simulink model "Example_AswarmTriangleCallibration"  (R2023b)
settings: Solver=FixedStepAuto  StartTime=0.0  StopTime=1  FixedStep=0.1  RelTol=1e-3  EnableMultiTasking=on
undefined symbols (not defined in the file or in its folder): numtestpoint4, testpoint4
libraries: simulink x1
settings Model: Creator=damerius  LastModifiedBy=khalis
settings SolverCC: ConcurrentTasks=on  AlgebraicLoopSolver=TrustRegion  PositivePriorityOrder=on
settings DataIOCC: SaveOutput=off  SignalLogging=off  DSMLogging=off  SaveTime=off  ReturnWorkspaceOutputs=off
settings OptimizationCC: DefaultParameterBehavior=Inlined  ReuseModelBlockBuffer=off  ZeroExternalMemoryAtStartup=off  ZeroInternalMemoryAtStartup=off  SimCompilerOptimization=on
settings DebuggingCC: UnconnectedInputMsg=warning  UnconnectedOutputMsg=warning  UnconnectedLineMsg=warning
settings HardwareCC: ProdBitPerLong=64  ProdHWDeviceType=Intel->x86-64 (Linux 64)
settings ModelReferenceCC: EnableRefExpFcnMdlSchedulingChecks=on
settings SFSimCC: SimParseCustomCode=off  SimGenImportedTypeDefs=on  SimTargetLang=C++
settings RTWCC: GenCodeOnly=on  PackageGeneratedCodeAndArtifacts=on  PackageName=PackNGo  RTWVerbose=off  BuildConfiguration=Faster Runs  TargetLang=C++  DLArmComputeVersion=19.05
settings CodeAppCC: ForceParamTrailComments=on  MaxIdLength=95  MATLABSourceComments=on  UseSimReservedNames=on
settings GRTTargetCC: TargetLangStandard=C++11 (ISO)  GenerateFullHeader=off  MatFileLogging=off  CodeInterfacePackaging=C++ class

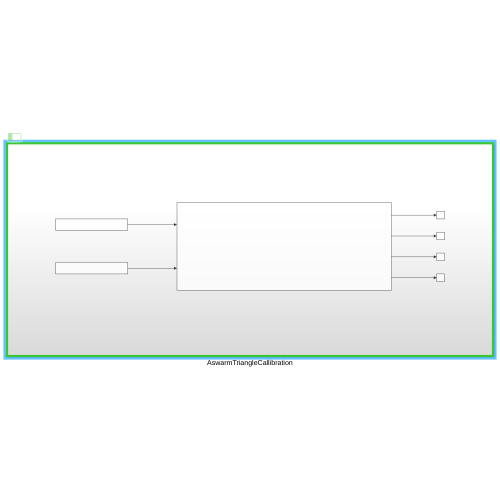
[thumbnail: Simulink's stored preview of the top-level diagram]
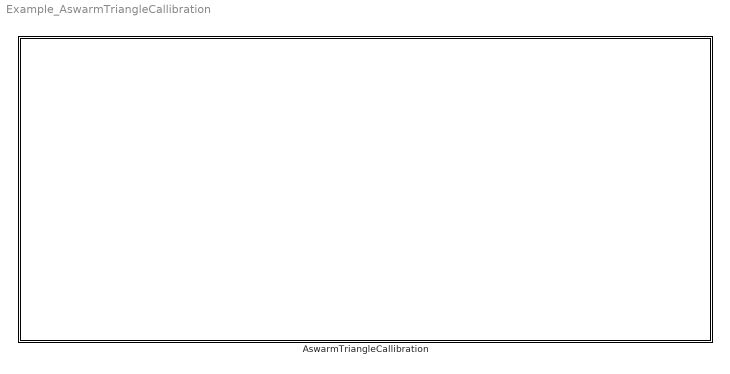
== system Example_AswarmTriangleCallibration ==
  AswarmTriangleCallibration : Subsystem  TreatAsAtomicUnit=on  ScheduleAs=Periodic partition  PartitionName=linedetector  SystemSampleTime=2

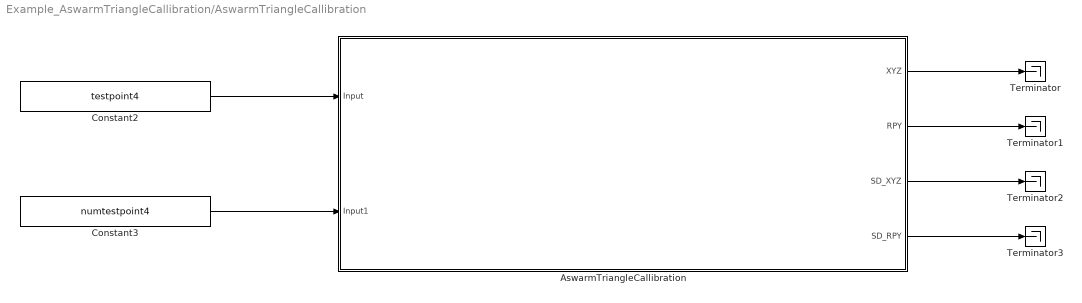
== system Example_AswarmTriangleCallibration/AswarmTriangleCallibration ==
  AswarmTriangleCallibration : Subsystem  ScheduleAs=Periodic partition  PartitionName=linedetector  SystemSampleTime=2  mask{Parameter1=0.1, Parameter2=1.0, Parameter3=500, Parameter4=256000, Parameter5=1.0, Parameter6=0.12, Parameter7=0.12, Parameter8=-2.0, Parameter9=-1.1, Parameter10=10.0, Parameter11=4.0, Parameter12=10.7703, Parameter13=90.0, Parameter14=21.80, Parameter15=68.20, Parameter16=0.001, Parameter17=0.001, Parameter18=2.0}
      mask prompts: Parameter1 "leafSize[m]:"; Parameter2 "clusterTolerance:"; Parameter3 "minClusterSize:"; Parameter4 "maxClusterSize:"; Parameter5 "radiusSearch[m]:"; Parameter6 "curvatureThresholdPlane:"; Parameter7 "curvatureThresholdCorner:"; Parameter8 "normalDistanceMin[m]:"; Parameter9 "normalDistanceMax[m]:"; Parameter10 "adjacentSide[m]:"; Parameter11 "oppositeSide[m]:"; Parameter12 "hypotenuse[m]:"; Parameter13 "adjacentAngle[°]:"; Parameter14 "oppositeAngle[°]:"; Parameter15 "vertexAngle[°]:"; Parameter16 "distanceTolerance[m]:"; Parameter17 "angleTolerance[°]:"; Parameter18 "searchRadius[m]:"
      mask DialogControl Container4 Prompt: Downsampling Parameter
      mask DialogControl Control2 Prompt: The size of the voxel grid for downsampling.
      mask DialogControl Container5 Prompt: Vehicle Clustering Parameter
      mask DialogControl Control3 Prompt: This algorithm will find nearest cluster as the vehicle cluster.
      mask DialogControl Container6 Prompt: Feature Extraction Parameter
      mask DialogControl Control4 Prompt: This algorithm will extract the plane and corner features.
      mask DialogControl Container9 Prompt: Plane Limit Parameter
      mask DialogControl Control5 Prompt: Sometime the vehicle surface plane is not visibile due to the object on the plane. Thus, to extract the surface plane only we need to apply passthrough filter in the plane normal.
      mask DialogControl Container10 Prompt: Ideal Triangle and Candidate Search Parameter:
      mask DialogControl Control7 Prompt: Ideal Right Triangle:
      mask DialogControl Control6 Prompt: This algorithm will find the best Right Triangle fit for the given input pointCloud.
      mask Display:
      | disp("Aswarm Triangle Callibration");
      | 
      | port_label('input',1,'inputCloud');
      | port_label('input',2,'numInputCloud');
  Constant2 : Constant  Value=testpoint4  OutDataTypeStr=single
  Constant3 : Constant  Value=numtestpoint4  OutDataTypeStr=uint32
  Terminator{,1..3} (4 alike) : Terminator
  wires:
  Constant2/1 -> AswarmTriangleCallibration/1(Input)
  Constant3/1 -> AswarmTriangleCallibration/2(Input1)
  AswarmTriangleCallibration/1(XYZ) -> Terminator/1
  AswarmTriangleCallibration/2(RPY) -> Terminator1/1
  AswarmTriangleCallibration/3(SD_XYZ) -> Terminator2/1
  AswarmTriangleCallibration/4(SD_RPY) -> Terminator3/1

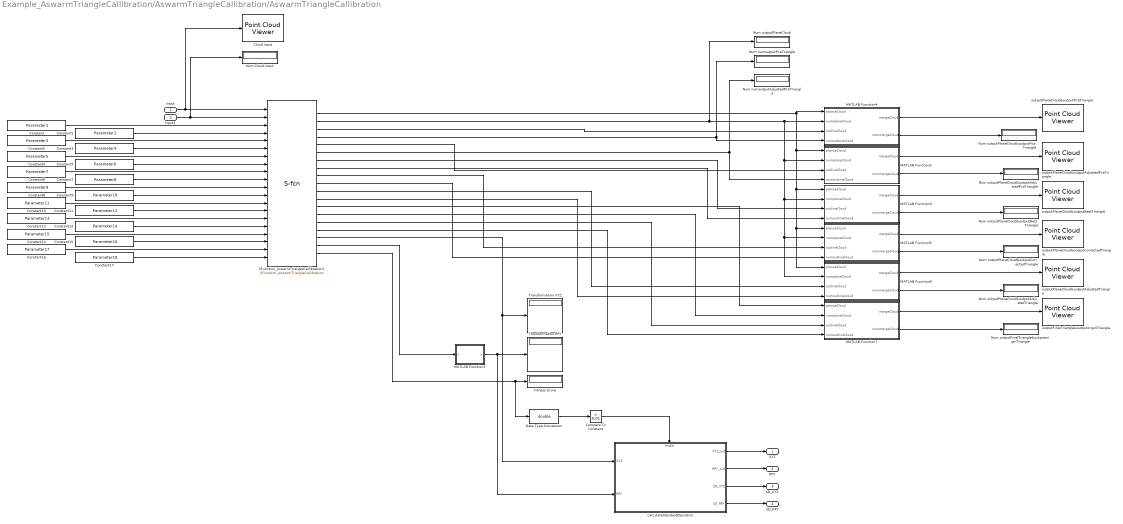
== system Example_AswarmTriangleCallibration/AswarmTriangleCallibration/AswarmTriangleCallibration ==
  Input : Inport
  Input1 : Inport  Port=2
  Cloud Input : PointCloudViewer  FigPos=[9 1380 570 1291]
  Compare To Constant : simulink/Logic and Bit Operations/Compare To Constant  relop=<  const=0.01  OutDataTypeStr=boolean
  Constant : Constant  Value=Parameter1  OutDataTypeStr=double
  Constant1 : Constant  Value=Parameter2  OutDataTypeStr=double
  Constant10 : Constant  Value=Parameter11  OutDataTypeStr=double
  Constant11 : Constant  Value=Parameter12  OutDataTypeStr=double
  Constant12 : Constant  Value=Parameter13  OutDataTypeStr=double
  Constant13 : Constant  Value=Parameter14  OutDataTypeStr=double
  Constant14 : Constant  Value=Parameter15  OutDataTypeStr=double
  Constant15 : Constant  Value=Parameter16  OutDataTypeStr=double
  Constant16 : Constant  Value=Parameter17  OutDataTypeStr=double
  Constant17 : Constant  Value=Parameter18  OutDataTypeStr=double
  Constant2 : Constant  Value=Parameter3  OutDataTypeStr=uint32
  Constant3 : Constant  Value=Parameter4  OutDataTypeStr=uint32
  Constant4 : Constant  Value=Parameter5  OutDataTypeStr=double
  Constant5 : Constant  Value=Parameter6  OutDataTypeStr=double
  Constant6 : Constant  Value=Parameter7  OutDataTypeStr=double
  Constant7 : Constant  Value=Parameter8  OutDataTypeStr=double
  Constant8 : Constant  Value=Parameter9  OutDataTypeStr=double
  Constant9 : Constant  Value=Parameter10  OutDataTypeStr=double
  Data Type Conversion : DataTypeConversion  OutDataTypeStr=double  SaturateOnIntegerOverflow=off  RndMeth=Floor
  Fitness Score : Display
  MATLAB Function1 : MATLAB Function  TreatAsAtomicUnit=on
  MATLAB Function2 : MATLAB Function  TreatAsAtomicUnit=on
  MATLAB Function3 : MATLAB Function  TreatAsAtomicUnit=on
  MATLAB Function4 : MATLAB Function  TreatAsAtomicUnit=on
  MATLAB Function5 : MATLAB Function  TreatAsAtomicUnit=on
  MATLAB Function6 : MATLAB Function  TreatAsAtomicUnit=on
  MATLAB Function7 : MATLAB Function  TreatAsAtomicUnit=on
  Num Cloud Input : Display
  Num numoutputAdjustedPcaTriangle : Display
  Num numoutputPcaTriangle : Display
  Num outputFinalTriangle&outputoriginTriangle : Display
  Num outputPlaneCloud : Display
  Num outputPlaneCloud&outputAdjustedPcaTriangle : Display
  Num outputPlaneCloud&outputAdjustedTriangle : Display
  Num outputPlaneCloud&outputBestTriangle : Display
  Num outputPlaneCloud&outputCorrectedTriangle : Display
  Num outputPlaneCloud&outputPcaTriangle : Display
  SFunction_AswarmTriangleCallibration1 : S-Function  FunctionName=SFunction_AswarmTriangleCallibration  Parameters=SampleTime  SFunctionDeploymentMode=off  EnableBusSupport=off  mask(Legacy Function){SFunctionSpec=void OutputAswarmTriangleCallibration(single u1[256000][3], uint32 u2,double u3,double u4, uint32 u5, uint32 u6,double u7, double u8, double u9,double u10, double u11,double u12, double u13, double u14,double u15, double u16, double u17,double u18, double u19, double u20,single y1[256000][3], uint32 y2,single y3[256000][3], uint32 y4,single y5[256000][3], uint32 y6,single y7[256000][3], uint32 y8,single y9[256000][3], uint32 y10,single y11[256000][3], uint32 y12,single y13[256000][3], uint32 y14,single y15[256000][3], uint32 y16,single y17[3][1], single y18[3][1],single y19), SampleTime=-1, ShowSpec=off}
      mask prompts: SampleTime "Sample time (-1 for inherited):"; ShowSpec "Display function specification"
      mask help:
      | This block allows you to call the legacy functions specified by the following Legacy Code Tool definition:
      | def.SFunctionName = 'SFunction_AswarmTriangleCallibration';
      | def.OutputFcnSpec = 'void OutputAswarmTriangleCallibration(single u1[256000][3], uint32 u2,double u3,double u4, uint32 u5, uint32 u6,double u7, double u8, double u9,double u10, double u11,double u12, double u13, double u14,double u15, double u16, double u17,double u18, double u19, double u20,single y1[256000][3], uint32 y2,single y3[256000][3], uint32 y4,single y5[256000][3], uint32 y6,single y7[256000][3], uint32 y8,single y9[256000][3], uint32 y10,single y11[256000][3], uint32 y12,single y13[256000][3], uint32 y14,single y15[256000][3], uint32 y16,single y17[3][1], single y18[3][1],single y19)';
      | def.StartFcnSpec = 'void CreateAswarmTriangleCallibration()';
      | def.TerminateFcnSpec = 'void DeleteAswarmTriangleCallibration()';
      | def.HeaderFiles = {'AswarmTriangleCallibration.h'};
      | def.SourceFiles = {'AswarmTriangleCallibration.cpp'};
      | def.SampleTime = 'parameterized';
      | def.Options.useTlcWithAccel = false;
      mask Help: <p>This block was generated automatically by the Legacy Code Tool. For detailed help on this tool, call<a href="matlab:legacy_code('help')"> legacy_code('help')</a>.</p>
      mask Callback ShowSpec:
      | if strcmp(get_param(gcbh, 'ShowSpec'), 'on')
      |   set_param(gcbh, 'MaskDisplay', sprintf('fprintf(''%s'');', get_param(gcbh, 'SFunctionSpec')));
      | else
      |   set_param(gcbh, 'MaskDisplay', sprintf('fprintf(''%s'');', get_param(gcbh, 'FunctionName')));
      | end
      mask Display: fprintf('SFunction_AswarmTriangleCallibration');
  Transformation RPY : Display
  Transformation XYZ : Display
  calculateStandardDeviation : Subsystem
  outputFinalTriangle&outputoriginTriangle : PointCloudViewer  FigPos=[3744 1078 570 989]
  outputPlaneCloud&outputAdjustedPcaTriangle : PointCloudViewer  FigPos=[1181 1380 570 1291]
  outputPlaneCloud&outputAdjustedTriangle : PointCloudViewer  FigPos=[3154 1074 578 989]
  outputPlaneCloud&outputBestTriangle : PointCloudViewer  FigPos=[1767 1380 570 1291]
  outputPlaneCloud&outputCorrectedTriangle : PointCloudViewer  FigPos=[2572 1078 570 989]
  outputPlaneCloud&outputPcaTriangle : PointCloudViewer  FigPos=[595 1380 570 1291]
  XYZ : Outport
  RPY : Outport  Port=2
  SD_XYZ : Outport  Port=3
  SD_RPY : Outport  Port=4
  wires:
  Constant/1 -> SFunction_AswarmTriangleCallibration1/3
  Input/1 -> SFunction_AswarmTriangleCallibration1/1, Cloud Input/1
  Input1/1 -> SFunction_AswarmTriangleCallibration1/2, Num Cloud Input/1
  Constant1/1 -> SFunction_AswarmTriangleCallibration1/4
  Constant2/1 -> SFunction_AswarmTriangleCallibration1/5
  Constant3/1 -> SFunction_AswarmTriangleCallibration1/6
  Constant4/1 -> SFunction_AswarmTriangleCallibration1/7
  Constant5/1 -> SFunction_AswarmTriangleCallibration1/8
  Constant6/1 -> SFunction_AswarmTriangleCallibration1/9
  Constant9/1 -> SFunction_AswarmTriangleCallibration1/12
  Constant10/1 -> SFunction_AswarmTriangleCallibration1/13
  Constant8/1 -> SFunction_AswarmTriangleCallibration1/11
  Constant11/1 -> SFunction_AswarmTriangleCallibration1/14
  Constant7/1 -> SFunction_AswarmTriangleCallibration1/10
  Constant12/1 -> SFunction_AswarmTriangleCallibration1/15
  Constant15/1 -> SFunction_AswarmTriangleCallibration1/18
  Constant16/1 -> SFunction_AswarmTriangleCallibration1/19
  Constant14/1 -> SFunction_AswarmTriangleCallibration1/17
  Constant17/1 -> SFunction_AswarmTriangleCallibration1/20
  Constant13/1 -> SFunction_AswarmTriangleCallibration1/16
  SFunction_AswarmTriangleCallibration1/17 -> Transformation XYZ/1, calculateStandardDeviation/1(XYZ)
  SFunction_AswarmTriangleCallibration1/19 -> Data Type Conversion/1, Fitness Score/1
  SFunction_AswarmTriangleCallibration1/18 -> MATLAB Function1/1(u)
  MATLAB Function1/1(y) -> Transformation RPY/1, calculateStandardDeviation/2(RPY)
  MATLAB Function4/2(nummergeCloud) -> Num outputPlaneCloud&outputPcaTriangle/1
  MATLAB Function4/1(mergeCloud) -> outputPlaneCloud&outputPcaTriangle/1
  MATLAB Function2/2(nummergeCloud) -> Num outputPlaneCloud&outputAdjustedPcaTriangle/1
  MATLAB Function2/1(mergeCloud) -> outputPlaneCloud&outputAdjustedPcaTriangle/1
  MATLAB Function3/2(nummergeCloud) -> Num outputPlaneCloud&outputBestTriangle/1
  MATLAB Function3/1(mergeCloud) -> outputPlaneCloud&outputBestTriangle/1
  MATLAB Function5/2(nummergeCloud) -> Num outputPlaneCloud&outputCorrectedTriangle/1
  MATLAB Function5/1(mergeCloud) -> outputPlaneCloud&outputCorrectedTriangle/1
  SFunction_AswarmTriangleCallibration1/1 -> MATLAB Function6/1(planceCloud), MATLAB Function5/1(planceCloud), MATLAB Function3/1(planceCloud), MATLAB Function2/1(planceCloud), MATLAB Function4/1(planceCloud)
  SFunction_AswarmTriangleCallibration1/2 -> MATLAB Function6/2(numplaneCloud), MATLAB Function5/2(numplaneCloud), MATLAB Function3/2(numplaneCloud), MATLAB Function2/2(numplaneCloud), MATLAB Function4/2(numplaneCloud), Num outputPlaneCloud/1
  SFunction_AswarmTriangleCallibration1/3 -> MATLAB Function4/3(outlineCloud)
  SFunction_AswarmTriangleCallibration1/4 -> MATLAB Function4/4(numoutlineCloud), Num numoutputPcaTriangle/1
  SFunction_AswarmTriangleCallibration1/5 -> MATLAB Function2/3(outlineCloud)
  SFunction_AswarmTriangleCallibration1/6 -> MATLAB Function2/4(numoutlineCloud), Num numoutputAdjustedPcaTriangle/1
  SFunction_AswarmTriangleCallibration1/7 -> MATLAB Function3/3(outlineCloud)
  SFunction_AswarmTriangleCallibration1/8 -> MATLAB Function3/4(numoutlineCloud)
  SFunction_AswarmTriangleCallibration1/9 -> MATLAB Function5/3(outlineCloud)
  SFunction_AswarmTriangleCallibration1/10 -> MATLAB Function5/4(numoutlineCloud)
  SFunction_AswarmTriangleCallibration1/11 -> MATLAB Function6/3(outlineCloud)
  SFunction_AswarmTriangleCallibration1/12 -> MATLAB Function6/4(numoutlineCloud)
  SFunction_AswarmTriangleCallibration1/13 -> MATLAB Function7/1(planceCloud)
  SFunction_AswarmTriangleCallibration1/14 -> MATLAB Function7/2(numplaneCloud)
  SFunction_AswarmTriangleCallibration1/15 -> MATLAB Function7/3(outlineCloud)
  SFunction_AswarmTriangleCallibration1/16 -> MATLAB Function7/4(numoutlineCloud)
  MATLAB Function6/2(nummergeCloud) -> Num outputPlaneCloud&outputAdjustedTriangle/1
  MATLAB Function6/1(mergeCloud) -> outputPlaneCloud&outputAdjustedTriangle/1
  MATLAB Function7/2(nummergeCloud) -> Num outputFinalTriangle&outputoriginTriangle/1
  MATLAB Function7/1(mergeCloud) -> outputFinalTriangle&outputoriginTriangle/1
  Compare To Constant/1 -> calculateStandardDeviation/Enable
  calculateStandardDeviation/1(XYZ_out) -> XYZ/1
  calculateStandardDeviation/2(RPY_out) -> RPY/1
  calculateStandardDeviation/3(SD_XYZ) -> SD_XYZ/1
  calculateStandardDeviation/4(SD_RPY) -> SD_RPY/1
  Data Type Conversion/1 -> Compare To Constant/1

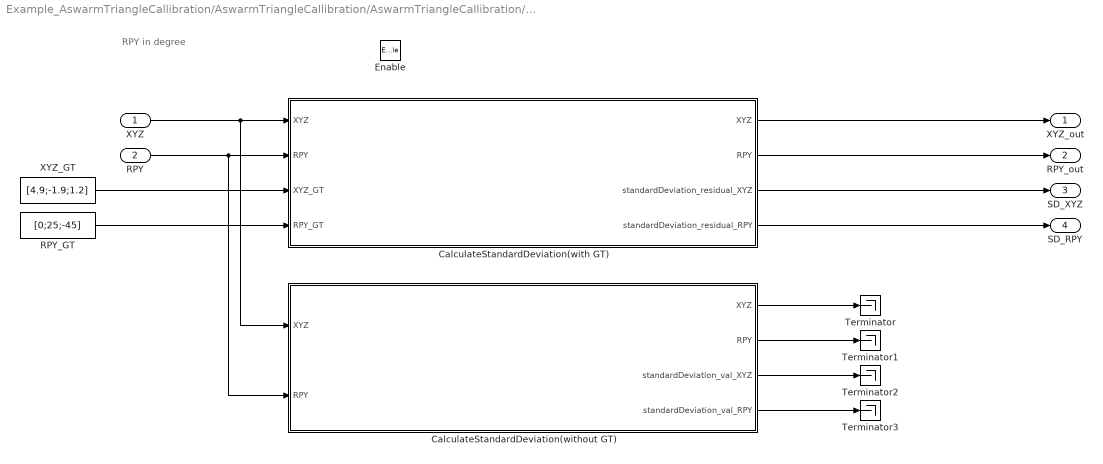
== system Example_AswarmTriangleCallibration/AswarmTriangleCallibration/AswarmTriangleCallibration/calculateStandardDeviation ==
  note: RPY in degree
  XYZ : Inport
  RPY : Inport  Port=2
  Enable : EnablePort
  CalculateStandardDeviation(with GT) : MATLAB Function  TreatAsAtomicUnit=on
  CalculateStandardDeviation(without GT) : MATLAB Function  TreatAsAtomicUnit=on
  RPY_GT : Constant  Value=[0;25;-45]
  Terminator{,1..3} (4 alike) : Terminator
  XYZ_GT : Constant  Value=[4.9;-1.9;1.2]
  XYZ_out : Outport
  RPY_out : Outport  Port=2
  SD_XYZ : Outport  Port=3
  SD_RPY : Outport  Port=4
  wires:
  XYZ/1 -> CalculateStandardDeviation(without GT)/1("XYZ "), CalculateStandardDeviation(with GT)/1("XYZ ")
  RPY/1 -> CalculateStandardDeviation(without GT)/2("RPY "), CalculateStandardDeviation(with GT)/2("RPY ")
  CalculateStandardDeviation(with GT)/1(XYZ) -> XYZ_out/1
  CalculateStandardDeviation(with GT)/2(RPY) -> RPY_out/1
  CalculateStandardDeviation(with GT)/3(standardDeviation_residual_XYZ) -> SD_XYZ/1
  CalculateStandardDeviation(with GT)/4(standardDeviation_residual_RPY) -> SD_RPY/1
  XYZ_GT/1 -> CalculateStandardDeviation(with GT)/3(XYZ_GT)
  RPY_GT/1 -> CalculateStandardDeviation(with GT)/4(RPY_GT)
  CalculateStandardDeviation(without GT)/1(XYZ) -> Terminator/1
  CalculateStandardDeviation(without GT)/2(RPY) -> Terminator1/1
  CalculateStandardDeviation(without GT)/3(standardDeviation_val_XYZ) -> Terminator2/1
  CalculateStandardDeviation(without GT)/4(standardDeviation_val_RPY) -> Terminator3/1

== matlab function Example_AswarmTriangleCallibration/AswarmTriangleCallibration/AswarmTriangleCallibration/MATLAB Function2 ==
  data: planceCloud input; mergeCloud output; numplaneCloud input; outlineCloud input; numoutlineCloud input; nummergeCloud output
function [mergeCloud, nummergeCloud] = fcn(planceCloud, numplaneCloud, outlineCloud, numoutlineCloud)

mergeCloud = NaN(2*(128*2000),3,'single');
nummergeCloud = numplaneCloud + numoutlineCloud;
if nummergeCloud< uint32(128*2000)
    mergeCloud(1:numplaneCloud,1:3) = planceCloud(1:numplaneCloud,1:3);
    offset= numplaneCloud + uint32(1);
    endset=numplaneCloud + numoutlineCloud;
    mergeCloud(offset:endset,1:3)  = outlineCloud(1:numoutlineCloud,1:3);
end

== matlab function Example_AswarmTriangleCallibration/AswarmTriangleCallibration/AswarmTriangleCallibration/MATLAB Function3 ==
  data: planceCloud input; mergeCloud output; numplaneCloud input; outlineCloud input; numoutlineCloud input; nummergeCloud output
function [mergeCloud, nummergeCloud] = fcn(planceCloud, numplaneCloud, outlineCloud, numoutlineCloud)

mergeCloud = NaN(2*(128*2000),3,'single');
nummergeCloud = numplaneCloud + numoutlineCloud;
if nummergeCloud< uint32(128*2000)
    mergeCloud(1:numplaneCloud,1:3) = planceCloud(1:numplaneCloud,1:3);
    offset= numplaneCloud + uint32(1);
    endset=numplaneCloud + numoutlineCloud;
    mergeCloud(offset:endset,1:3)  = outlineCloud(1:numoutlineCloud,1:3);
end

== matlab function Example_AswarmTriangleCallibration/AswarmTriangleCallibration/AswarmTriangleCallibration/MATLAB Function5 ==
  data: planceCloud input; mergeCloud output; numplaneCloud input; outlineCloud input; numoutlineCloud input; nummergeCloud output
function [mergeCloud, nummergeCloud] = fcn(planceCloud, numplaneCloud, outlineCloud, numoutlineCloud)

mergeCloud = NaN(2*(128*2000),3,'single');
nummergeCloud = numplaneCloud + numoutlineCloud;
if nummergeCloud< uint32(128*2000)
    mergeCloud(1:numplaneCloud,1:3) = planceCloud(1:numplaneCloud,1:3);
    offset= numplaneCloud + uint32(1);
    endset=numplaneCloud + numoutlineCloud;
    mergeCloud(offset:endset,1:3)  = outlineCloud(1:numoutlineCloud,1:3);
end

== matlab function Example_AswarmTriangleCallibration/AswarmTriangleCallibration/AswarmTriangleCallibration/MATLAB Function6 ==
  data: planceCloud input; mergeCloud output; numplaneCloud input; outlineCloud input; numoutlineCloud input; nummergeCloud output
function [mergeCloud, nummergeCloud] = fcn(planceCloud, numplaneCloud, outlineCloud, numoutlineCloud)

mergeCloud = NaN(2*(128*2000),3,'single');
nummergeCloud = numplaneCloud + numoutlineCloud;
if nummergeCloud< uint32(128*2000)
    mergeCloud(1:numplaneCloud,1:3) = planceCloud(1:numplaneCloud,1:3);
    offset= numplaneCloud + uint32(1);
    endset=numplaneCloud + numoutlineCloud;
    mergeCloud(offset:endset,1:3)  = outlineCloud(1:numoutlineCloud,1:3);
end

== matlab function Example_AswarmTriangleCallibration/AswarmTriangleCallibration/AswarmTriangleCallibration/MATLAB Function7 ==
  data: planceCloud input; mergeCloud output; numplaneCloud input; outlineCloud input; numoutlineCloud input; nummergeCloud output
function [mergeCloud, nummergeCloud] = fcn(planceCloud, numplaneCloud, outlineCloud, numoutlineCloud)

mergeCloud = NaN(128*2000,3,'single');
nummergeCloud = numplaneCloud + numoutlineCloud;
if nummergeCloud< uint32(128*2000)
    mergeCloud(1:numplaneCloud,1:3) = planceCloud(1:numplaneCloud,1:3);
    offset= numplaneCloud + uint32(1);
    endset=numplaneCloud + numoutlineCloud;
    mergeCloud(offset:endset,1:3)  = outlineCloud(1:numoutlineCloud,1:3);
end

== matlab function Example_AswarmTriangleCallibration/AswarmTriangleCallibration/AswarmTriangleCallibration/MATLAB Function1 ==
  data: u input; y output
function y = fcn(u)

y = rad2deg(u);

== matlab function Example_AswarmTriangleCallibration/AswarmTriangleCallibration/AswarmTriangleCallibration/MATLAB Function4 ==
  data: planceCloud input; mergeCloud output; numplaneCloud input; outlineCloud input; numoutlineCloud input; nummergeCloud output
function [mergeCloud, nummergeCloud] = fcn(planceCloud, numplaneCloud, outlineCloud, numoutlineCloud)

mergeCloud = NaN(128*2000,3,'single');
nummergeCloud = numplaneCloud + numoutlineCloud;
if nummergeCloud< uint32(128*2000)
    mergeCloud(1:numplaneCloud,1:3) = planceCloud(1:numplaneCloud,1:3);
    offset= numplaneCloud + uint32(1);
    endset=numplaneCloud + numoutlineCloud;
    mergeCloud(offset:endset,1:3)  = outlineCloud(1:numoutlineCloud,1:3);
end

== matlab function Example_AswarmTriangleCallibration/AswarmTriangleCallibration/AswarmTriangleCallibration/calculateStandardDeviation/CalculateStandardDeviation(without GT) ==
  data: XYZ input; XYZ output; RPY input; RPY output; standardDeviation_val_XYZ output; standardDeviation_val_RPY output
function [XYZ,RPY,standardDeviation_val_XYZ,standardDeviation_val_RPY] = computeUncertainties(XYZ,RPY)  
    itrSize = uint32(10);
    persistent val_RPY; if(isempty(val_RPY)), val_RPY = zeros(3,itrSize); end
    persistent val_XYZ; if(isempty(val_XYZ)), val_XYZ = zeros(3,itrSize); end
    persistent counter; if(isempty(counter)), counter = uint32(0); end

    if counter == uint32(itrSize)
        counter = counter - uint32(1);
        val_XYZ(1:3,1:4) = val_XYZ(1:3,2:5);
        val_RPY(1:3,1:4) = val_RPY(1:3,2:5);
    end
    if counter < uint32(itrSize)
        counter = counter  + uint32(1);
        val_XYZ(1:3,counter) = XYZ(1:3,1);
        val_RPY(1:3,counter) = RPY(1:3,1);
    end

    mean_val_XYZ = calculateMean(val_XYZ,counter);
    mean_val_RPY = calculateMean(val_RPY,counter);

    variance_val_XYZ = calculateVariance(val_XYZ,mean_val_XYZ,counter);
    variance_val_RPY = calculateVariance(val_RPY,mean_val_RPY,counter);

    standardDeviation_val_XYZ = sqrt(variance_val_XYZ);
    standardDeviation_val_RPY = sqrt(variance_val_RPY);

end

function meanVal = calculateMean(val,size)
    cum= zeros(3,1);
    size = double(size);
    for i = 1:size
        cum = cum + val(:,i);
    end
    meanVal = cum./size;
end

function variance = calculateVariance(val, meanval, size)
    variance = zeros(3,1);  % Initialize variance as a column vector with three elements
    size = double(size);
    for i = 1:size
        variance = variance + (val(1:3,i) - meanval).^2;  % Accumulate squared deviations
    end
    variance = variance ./ size;  % Divide by the number of elements to get the average
end

== matlab function Example_AswarmTriangleCallibration/AswarmTriangleCallibration/AswarmTriangleCallibration/calculateStandardDeviation/CalculateStandardDeviation(with GT) ==
  data: XYZ input; XYZ output; RPY input; RPY output; standardDeviation_residual_XYZ output; XYZ_GT input; RPY_GT input; standardDeviation_residual_RPY output
function [XYZ,RPY,standardDeviation_residual_XYZ,standardDeviation_residual_RPY] = computeUncertainties(XYZ,RPY,XYZ_GT,RPY_GT)
    itrSize = uint32(10);
    persistent residual_RPY; if(isempty(residual_RPY)), residual_RPY = zeros(3,itrSize); end
    persistent residual_XYZ; if(isempty(residual_XYZ)), residual_XYZ = zeros(3,itrSize); end
    persistent counter; if(isempty(counter)), counter = uint32(0); end

    if counter == uint32(itrSize)
        counter = counter - uint32(1);
        residual_XYZ(1:3,1:4) = residual_XYZ(1:3,2:5);
        residual_RPY(1:3,1:4) = residual_RPY(1:3,2:5);
    end
    if counter < uint32(itrSize)
        counter = counter  + uint32(1);
        residual_XYZ(1:3,counter) = XYZ(1:3,1)-XYZ_GT(1:3,1);
        residual_RPY(1:3,counter) = RPY(1:3,1)-RPY_GT(1:3,1);
    end

    mean_residual_XYZ = calculateMean(residual_XYZ,counter);
    mean_residual_RPY = calculateMean(residual_RPY,counter);

    variance_residual_XYZ = calculateVariance(residual_XYZ,mean_residual_XYZ,counter);
    variance_residual_RPY = calculateVariance(residual_RPY,mean_residual_RPY,counter);

    standardDeviation_residual_XYZ = sqrt(variance_residual_XYZ);
    standardDeviation_residual_RPY = sqrt(variance_residual_RPY);

end

function meanVal = calculateMean(val,size)
    cum= zeros(3,1);
    size = double(size);
    for i = 1:size
        cum = cum + val(:,i);
    end
    meanVal = cum./size;
end

function variance = calculateVariance(val, meanval, size)
    variance = zeros(3,1);  % Initialize variance as a column vector with three elements
    size = double(size);
    for i = 1:size
        variance = variance + (val(1:3,i) - meanval).^2;  % Accumulate squared deviations
    end
    variance = variance ./ size;  % Divide by the number of elements to get the average
end
